simulink model "DatosIdentN20Suelo"  (R2025a)
settings: Solver=FixedStepDiscrete  StartTime=0.0  StopTime=10  FixedStep=0.01  RelTol=1e-3  EnableMultiTasking=on
libraries: SignalEditorBlockLib x1, arduinowifilib x1
settings Model: SILPILModeSetting=veronly  ExtModeTrigDuration=2  Creator=Antonio  LastModifiedBy=aj
settings SolverCC: AutoInsertRateTranBlk=on
settings OptimizationCC: EnhancedBackFolding=on  PassReuseOutputArgsAs=Individual arguments  ZeroExternalMemoryAtStartup=off  ZeroInternalMemoryAtStartup=off  MaxStackSize=64  OptimizeBlockOrder=speed  DifferentSizesBufferReuse=on  OptimizationCustomize=off  EfficientTunableParamExpr=on
settings DebuggingCC: ParameterTunabilityLossMsg=error
settings HardwareCC: ProdBitPerPointer=32.0  ProdBitPerSizeT=32.0  ProdBitPerPtrDiffT=32.0  ProdLargestAtomicInteger=Long  ProdLargestAtomicFloat=Double  ProdWordSize=32.0  ProdHWDeviceType=ARM Compatible->ARM Cortex
settings SFSimCC: MATLABDynamicMemAlloc=off
settings RTWCC: SystemTargetFile=ert.tlc  HardwareBoard=ESP32-WROOM (Arduino Compatible)  TLCOptions="-aInlineSetEventsForThisBaseRateFcn=TLC_FALSE -aSuppressMultiTaskScheduler=TLC_FALSE  -aRateBasedStepFcn=0"  TemplateMakefile=ert_default_tmf  Toolchain=ESP32  BuildConfiguration=Faster Runs  GPUComputeCapability=3.5  Description=Embedded Coder
settings CodeAppCC: ForceParamTrailComments=on  IgnoreCustomStorageClasses=off  OperatorAnnotations=on  SimulinkDataObjDesc=on  SFDataObjDesc=on  InsertBlockDesc=on
settings ERTTargetCC: ExtModeTransport=3.0  ExtModeAutomaticAllocSize=off  ExtModeStaticAllocSize=65536.0  InlinedParameterPlacement=Hierarchical  DynamicArrayContainerType=coder::array  SupportContinuousTime=on  SupportVariableSizeSignals=on

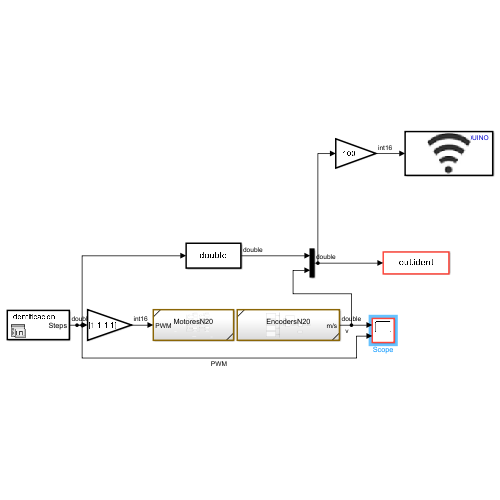
[thumbnail: Simulink's stored preview of the top-level diagram]
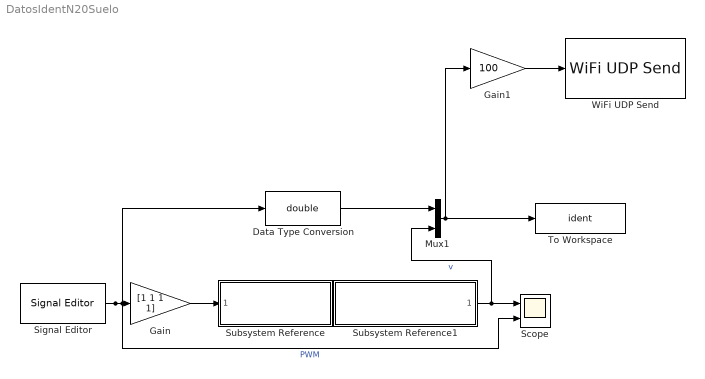
== system DatosIdentN20Suelo ==
  Data Type Conversion : DataTypeConversion  OutDataTypeStr=double  SaturateOnIntegerOverflow=off  RndMeth=Floor
  Gain : Gain  Gain=[1 1 1 1]  OutDataTypeStr=int16
  Gain1 : Gain  Gain=100  OutDataTypeStr=int16
  Mux1 : Mux  Inputs=2
  Scope : Scope  NumInputPorts=2
      settings: ActiveDisplayYMinimum=-0.87381155657908494  ActiveDisplayYMaximum=0.86304038176763243
  Signal Editor : SignalEditorBlockLib/Signal Editor  FileName=Rampa.mat  ActiveScenario=Identificacion  ActiveSignal=Steps  IsBus=off  OutputBusObjectStr=Bus: BusObject  SampleTime=0  Interpolate=off  ZeroCross=off  OutputAfterFinalValue=Setting to zero  Unit=inherit  PreserveSignalName=on  ApplySigPropsToAllScenarios=on  ApplySigPropsToAllSignals=off  SignalPropertySource=Dialog parameters
  Subsystem Reference : Subsystem  ReferencedSubsystem=MotoresN20
  Subsystem Reference1 : Subsystem  ReferencedSubsystem=EncodersN20
  To Workspace : ToWorkspace  VariableName=ident  SampleTime=-1
      settings: Save2DSignal=2-D array (concatenate along first dimension)
  WiFi UDP Send : arduinowifilib/WiFi UDP Send  remoteIPOctetString=192.168.137.1  remoteport=55002  localport=55001  remoteipoctet1=192  remoteipoctet2=168  remoteipoctet3=137  remoteipoctet4=1  wifiUDPIndex=0  blockPlatform=ARDUINO  isARMArch=false
  wires:
  Signal Editor/1 -> Scope/2, Data Type Conversion/1, Gain/1  "PWM"
  Subsystem Reference1/1 -> Mux1/2, Scope/1  "v"
  Mux1/1 -> Gain1/1, To Workspace/1
  Data Type Conversion/1 -> Mux1/1
  Gain/1 -> Subsystem Reference/1
  Gain1/1 -> WiFi UDP Send/1
